simulink model "IntakeManifold_Model"  (R2024b)
settings: Solver=ode45  StartTime=0.0  StopTime=5  RelTol=1e-3
settings Model: Creator=viviankaspar  LastModifiedBy=viviankaspar

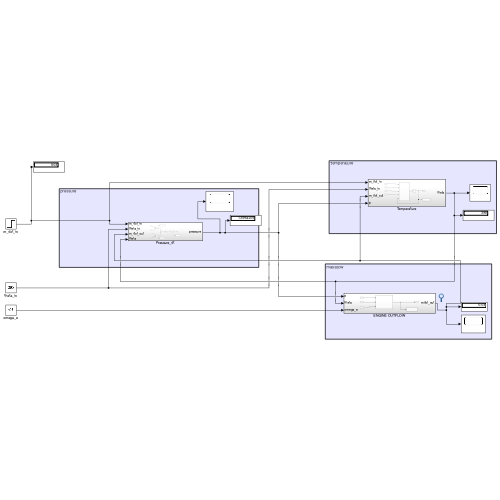
[thumbnail: Simulink's stored preview of the top-level diagram]
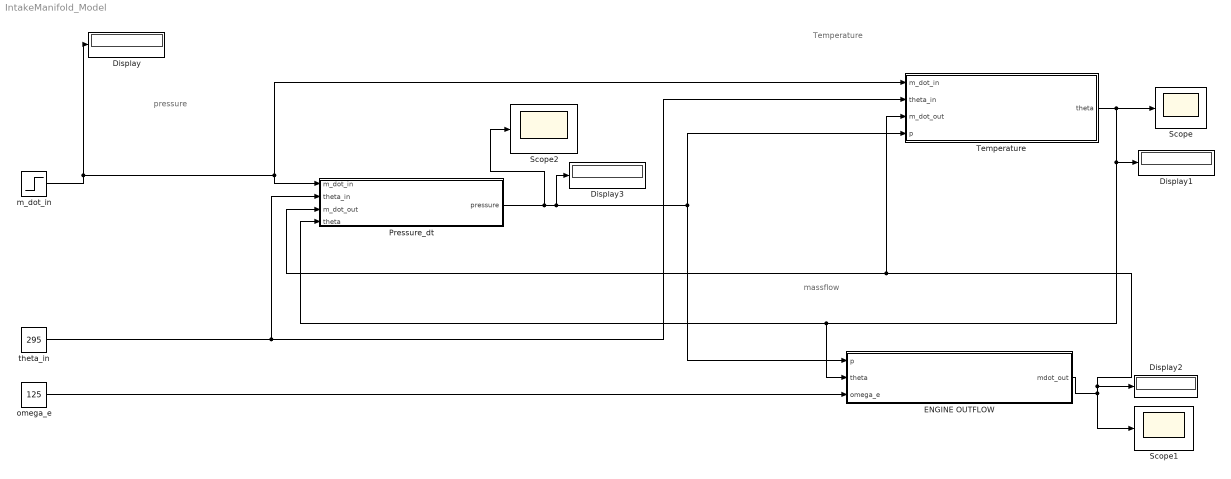
== system IntakeManifold_Model ==
  note: Temperature
  note: massflow
  note: pressure
  Display{,1..3} (4 alike) : Display
  ENGINE OUTFLOW : Subsystem
  Pressure_dt : Subsystem
  Scope : Scope
  Scope1 : Scope
  Scope2 : Scope
  Temperature : Subsystem
  m_dot_in : Step  Time=0.2  Before=0.02  After=0.03  SampleTime=0
  omega_e : Constant  Value=125
  theta_in : Constant  Value=295
  wires:
  Pressure_dt/1(pressure) -> Scope2/1, Display3/1, ENGINE OUTFLOW/1(p), Temperature/4(p)
  Temperature/1(theta) -> Display1/1, Pressure_dt/4(theta), ENGINE OUTFLOW/2(theta), Scope/1
  omega_e/1 -> ENGINE OUTFLOW/3(omega_e)
  ENGINE OUTFLOW/1(mdot_out) -> Display2/1, Pressure_dt/3(m_dot_out), Temperature/3(m_dot_out), Scope1/1
  m_dot_in/1 -> Display/1, Pressure_dt/1(m_dot_in), Temperature/1(m_dot_in)
  theta_in/1 -> Temperature/2(theta_in), Pressure_dt/2(theta_in)

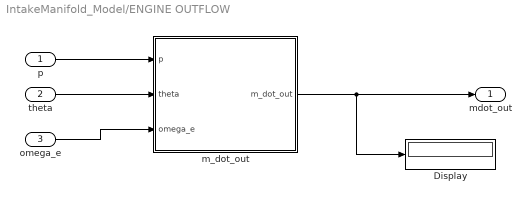
== system IntakeManifold_Model/ENGINE OUTFLOW ==
  p : Inport
  theta : Inport  Port=2
  omega_e : Inport  Port=3
  Display : Display
  m_dot_out : MATLAB Function  TreatAsAtomicUnit=on  mask{Vd=2.5*10^-3, kappa=1003/717, R=287, epsilon=10, pe=10^5, lambda_lw=0.8}
  mdot_out : Outport
  wires:
  p/1 -> m_dot_out/1(p)
  theta/1 -> m_dot_out/2(theta)
  omega_e/1 -> m_dot_out/3(omega_e)
  m_dot_out/1(m_dot_out) -> Display/1, mdot_out/1

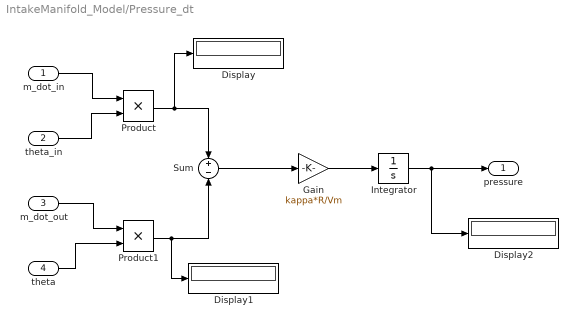
== system IntakeManifold_Model/Pressure_dt ==
  m_dot_in : Inport
  theta_in : Inport  Port=2
  m_dot_out : Inport  Port=3
  theta : Inport  Port=4
  Display : Display
  Display1 : Display
  Display2 : Display
  Gain : Gain  Gain=kappa*R/Vm  mask{kappa=1003/717, R=287, Vm=7.5*10^-3}
  Integrator : Integrator  InitialCondition=10^5  LimitOutput=on  UpperSaturationLimit=5e6
  Product : Product
  Product1 : Product
  Sum : Sum  Inputs=+-
  pressure : Outport
  wires:
  m_dot_in/1 -> Product/1
  theta_in/1 -> Product/2
  m_dot_out/1 -> Product1/1
  theta/1 -> Product1/2
  Product/1 -> Display/1, Sum/1
  Product1/1 -> Display1/1, Sum/2
  Sum/1 -> Gain/1
  Gain/1 -> Integrator/1
  Integrator/1 -> Display2/1, pressure/1

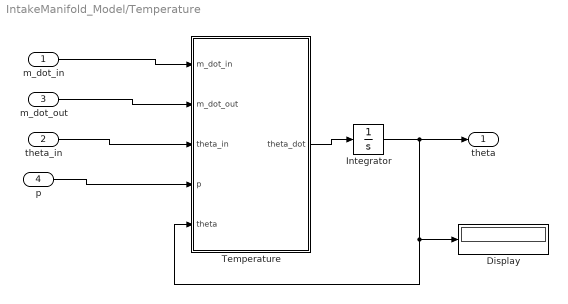
== system IntakeManifold_Model/Temperature ==
  m_dot_in : Inport
  theta_in : Inport  Port=2
  m_dot_out : Inport  Port=3
  p : Inport  Port=4
  " Temperature" : MATLAB Function  TreatAsAtomicUnit=on  mask{R=287, Vm=7.5*10^-3, Cv=717, Cp=1003}
  Display : Display
  Integrator : Integrator  InitialCondition=295
  theta : Outport
  wires:
  m_dot_out/1 -> " Temperature"/2(m_dot_out)
  " Temperature"/1(theta_dot) -> Integrator/1
  Integrator/1 -> Display/1, " Temperature"/5(theta), theta/1
  p/1 -> " Temperature"/4(p)
  m_dot_in/1 -> " Temperature"/1(m_dot_in)
  theta_in/1 -> " Temperature"/3(theta_in)

== matlab function IntakeManifold_Model/ENGINE OUTFLOW/m_dot_out ==
  data: p input; m_dot_out output; theta input; omega_e input; Vd parameter; kappa parameter; R parameter; pe parameter; lambda_lw parameter; epsilon parameter
function m_dot_out = fcn(p,theta,omega_e, Vd, kappa, R, pe, lambda_lw, epsilon)

m_dot_out = p/(R*theta)*Vd*omega_e/(4*pi)*lambda_lw*(epsilon/(epsilon-1)-1/(epsilon-1)*(pe/p)^(1/kappa));

== matlab function IntakeManifold_Model/Temperature/ Temperature ==
  data: m_dot_in input; m_dot_out input; theta_in input; p input; theta input; theta_dot output; Cv parameter; R parameter; Vm parameter; Cp parameter
function theta_dot = fcn(m_dot_in, m_dot_out, theta_in, p, theta, Cv, R, Vm, Cp)

theta_dot = theta*R/(p*Vm*Cv)*(Cp * (m_dot_in*theta_in-m_dot_out*theta)-Cv*(m_dot_in-m_dot_out)*theta);
